simulink model "Pump_system_008"  (R2020a)
settings: Solver=VariableStepAuto  StartTime=0.0  StopTime=1000  MaxStep=0.5  RelTol=1e-3  AbsTol=1e-4
libraries: subsea_lib x65, nesl_utility x44
(part 1 of 2)
settings Model: PauseTimes=645  EnablePacing=on  Creator=piosi  LastModifiedBy=piosi
settings SolverCC: AutoScaleAbsTol=off  MaxOrder=2  MaxConsecutiveZCs=10  MaxConsecutiveMinStep=2  ZeroCrossControl=EnableAll  ZeroCrossAlgorithm=Adaptive
settings DebuggingCC: ReadBeforeWriteMsg=DisableAll  WriteAfterWriteMsg=DisableAll  WriteAfterReadMsg=DisableAll  MultiTaskDSMMsg=none  SymbolicDimsDataTypeCodeGenerationDiagnostic=none
settings ModelReferenceCC: UpdateModelReferenceTargets=IfOutOfDate
settings SFSimCC: SFSimEcho=off  CustomCodeUndefinedFunction=UseInterfaceOnly
settings SimscapeCC: SimscapeLogType=all  SimscapeLogSimulationStatistics=on  SimscapeLogDataHistory=10000

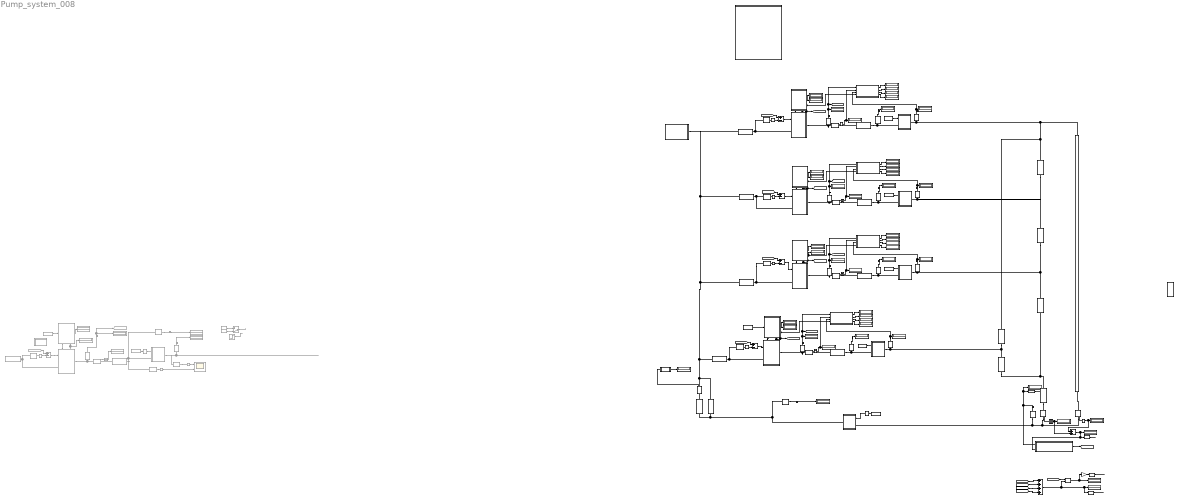
== system Pump_system_008 ==
  note: MANIFOLD
  note: PUMP 801
  note: 1. Find components in the Simscape library .
      | For more information, see Physical Modeling - Blocks .
      | 2. Connect the components to form a physical network.
      | For more information, see Essential Steps for Constructing a Physical Model .
      | 3. Explore simulation results using sscexplore
  note: Simscape Library Resources
  note: PUMP 802
  note: PUMP 803
  note: PUMP 805
  note: PUMP 805
  Add : Sum
  Add1 : Sum  Inputs=++++
  Butterfly valve Z011 : Subsystem
      mask Display: image('D:\CUvalley\Edycja 2\Dane katalogowe\Z-011.png'); % Use "Edit Image" on toolstrip to change.
  Butterfly valve Z1 : Subsystem
      mask Display: image('D:\CUvalley\Edycja 2\Dane katalogowe\Z-011.png'); % Use "Edit Image" on toolstrip to change.
  Butterfly valve Z2 : Subsystem
      mask Display: image('D:\CUvalley\Edycja 2\Dane katalogowe\Z-011.png'); % Use "Edit Image" on toolstrip to change.
  Butterfly valve Z4 : Subsystem
      mask Display: image('D:\CUvalley\Edycja 2\Dane katalogowe\Z-011.png'); % Use "Edit Image" on toolstrip to change.
  Butterfly valve Z5 : Subsystem  Commented=on
      mask Display: image('D:\CUvalley\Edycja 2\Dane katalogowe\Z-011.png'); % Use "Edit Image" on toolstrip to change.
  Constant1 : Constant  Commented=on  Value=0
  Constant2 : Constant  Commented=on
  Display{,1..17,19,21..40,43..51} (48 alike) : Display
      settings: Decimation=2
  Display{52..57} (6 alike) : Display  Commented=on
      settings: Decimation=2
  Divide : Product  Inputs=*/
  From7 : From  Commented=on  GotoTag=p_pump5
  Gain2 : Gain  Gain=100
  Goto10 : Goto  Commented=on  GotoTag=p_pump5
  Hydraulic Pipeline{1,4,10,13} (4 alike) : subsea_lib/Lines/Hydraulic Pipeline  ss_location=true  on_seabed=false  d_in=350 mm  D_out=370 mm  length=10 m  roughness=15e-6 m  Re_lam=2000  Re_turb=4000  wall_type=true  p_init=.101 bar  Young_modulus=5 GPa  time_const=0.01 s  k_sh=1.4
      settings: SourceProductName=Subsea  InternalSimscapePortConfiguration="{\"Bottom\":[],\"Left\":[{\"id\":\"A\",\"label\":\"A\",\"type\":\"subsea.ss_hydraulic\"}],\"Right\":[{\"id\":\"B\",\"label\":\"B\",\"type\":\"subsea.ss_hydraulic\"}],\"Top\":[]}"
  Hydraulic Pipeline{3,5,11,19} (4 alike) : subsea_lib/Lines/Hydraulic Pipeline  ss_location=true  on_seabed=false  d_in=300 mm  D_out=320 mm  length=2 m  roughness=15e-6 m  Re_lam=2000  Re_turb=4000  wall_type=true  p_init=0.1 bar  Young_modulus=195 GPa  time_const=0.01 s  k_sh=1.4
      settings: SourceProductName=Subsea  InternalSimscapePortConfiguration="{\"Bottom\":[],\"Left\":[{\"id\":\"A\",\"label\":\"A\",\"type\":\"subsea.ss_hydraulic\"}],\"Right\":[{\"id\":\"B\",\"label\":\"B\",\"type\":\"subsea.ss_hydraulic\"}],\"Top\":[]}"
  Hydraulic Pipeline12 : subsea_lib/Lines/Hydraulic Pipeline  Commented=on  ss_location=true  on_seabed=false  d_in=350 mm  D_out=370 mm  length=10 m  roughness=15e-6 m  Re_lam=2000  Re_turb=4000  wall_type=true  p_init=.101 bar  Young_modulus=5 GPa  time_const=0.01 s  k_sh=1.4
      settings: SourceProductName=Subsea  InternalSimscapePortConfiguration="{\"Bottom\":[],\"Left\":[{\"id\":\"A\",\"label\":\"A\",\"type\":\"subsea.ss_hydraulic\"}],\"Right\":[{\"id\":\"B\",\"label\":\"B\",\"type\":\"subsea.ss_hydraulic\"}],\"Top\":[]}"
  Hydraulic Pipeline14 : subsea_lib/Lines/Hydraulic Pipeline  ss_location=true  on_seabed=false  d_in=500 mm  D_out=520 mm  length=150 m  roughness=15e-6 m  Re_lam=2000  Re_turb=4000  wall_type=true  p_init=0.1 bar  Young_modulus=6 GPa  time_const=0.01 s  k_sh=1.4
      settings: SourceProductName=Subsea  InternalSimscapePortConfiguration="{\"Bottom\":[],\"Left\":[{\"id\":\"A\",\"label\":\"A\",\"type\":\"subsea.ss_hydraulic\"}],\"Right\":[{\"id\":\"B\",\"label\":\"B\",\"type\":\"subsea.ss_hydraulic\"}],\"Top\":[]}"
  Hydraulic Pipeline15 : subsea_lib/Lines/Hydraulic Pipeline  Commented=on  ss_location=true  on_seabed=false  d_in=300 mm  D_out=320 mm  length=2 m  roughness=15e-6 m  Re_lam=2000  Re_turb=4000  wall_type=true  p_init=0.1 bar  Young_modulus=195 GPa  time_const=0.01 s  k_sh=1.4
      settings: SourceProductName=Subsea  InternalSimscapePortConfiguration="{\"Bottom\":[],\"Left\":[{\"id\":\"A\",\"label\":\"A\",\"type\":\"subsea.ss_hydraulic\"}],\"Right\":[{\"id\":\"B\",\"label\":\"B\",\"type\":\"subsea.ss_hydraulic\"}],\"Top\":[]}"
  Hydraulic Pipeline{6..7,16..17} (4 alike) : subsea_lib/Lines/Hydraulic Pipeline  ss_location=true  on_seabed=false  d_in=500 mm  D_out=520 mm  length=5 m  roughness=15e-6 m  Re_lam=2000  Re_turb=4000  wall_type=true  p_init=0.1 bar  Young_modulus=6 GPa  time_const=0.01 s  k_sh=1.4
      settings: SourceProductName=Subsea  InternalSimscapePortConfiguration="{\"Bottom\":[],\"Left\":[{\"id\":\"A\",\"label\":\"A\",\"type\":\"subsea.ss_hydraulic\"}],\"Right\":[{\"id\":\"B\",\"label\":\"B\",\"type\":\"subsea.ss_hydraulic\"}],\"Top\":[]}"
  Hydraulic Pipeline18 : subsea_lib/Lines/Hydraulic Pipeline  ss_location=true  on_seabed=false  d_in=500 mm  D_out=520 mm  length=20 m  roughness=15e-6 m  Re_lam=2000  Re_turb=4000  wall_type=true  p_init=0.1 bar  Young_modulus=6 GPa  time_const=0.01 s  k_sh=1.4
      settings: SourceProductName=Subsea  InternalSimscapePortConfiguration="{\"Bottom\":[],\"Left\":[{\"id\":\"A\",\"label\":\"A\",\"type\":\"subsea.ss_hydraulic\"}],\"Right\":[{\"id\":\"B\",\"label\":\"B\",\"type\":\"subsea.ss_hydraulic\"}],\"Top\":[]}"
  Hydraulic Pipeline2 : subsea_lib/Lines/Hydraulic Pipeline  ss_location=true  on_seabed=false  d_in=500 mm  D_out=520 mm  length=10 m  roughness=15e-6 m  Re_lam=2000  Re_turb=4000  wall_type=true  p_init=0.1 bar  Young_modulus=6 GPa  time_const=0.01 s  k_sh=1.4
      settings: SourceProductName=Subsea  InternalSimscapePortConfiguration="{\"Bottom\":[],\"Left\":[{\"id\":\"A\",\"label\":\"A\",\"type\":\"subsea.ss_hydraulic\"}],\"Right\":[{\"id\":\"B\",\"label\":\"B\",\"type\":\"subsea.ss_hydraulic\"}],\"Top\":[]}"
  Hydraulic Pipeline20 : subsea_lib/Lines/Hydraulic Pipeline  ss_location=true  on_seabed=false  d_in=500 mm  D_out=520 mm  length=20 m  roughness=15e-6 m  Re_lam=2000  Re_turb=4000  wall_type=true  p_init=0.1 bar  Young_modulus=6 GPa  time_const=0.01 s  k_sh=1.4
      settings: SourceProductName=Subsea  InternalSimscapePortConfiguration="{\"Bottom\":[],\"Left\":[{\"id\":\"A\",\"label\":\"A\",\"type\":\"subsea.ss_hydraulic\"}],\"Right\":[{\"id\":\"B\",\"label\":\"B\",\"type\":\"subsea.ss_hydraulic\"}],\"Top\":[]}"
  Hydraulic Pipeline8 : subsea_lib/Lines/Hydraulic Pipeline  ss_location=true  on_seabed=false  d_in=500 mm  D_out=520 mm  length=30 m  roughness=15e-6 m  Re_lam=2000  Re_turb=4000  wall_type=true  p_init=0.1 bar  Young_modulus=6 GPa  time_const=0.01 s  k_sh=1.4
      settings: SourceProductName=Subsea  InternalSimscapePortConfiguration="{\"Bottom\":[],\"Left\":[{\"id\":\"A\",\"label\":\"A\",\"type\":\"subsea.ss_hydraulic\"}],\"Right\":[{\"id\":\"B\",\"label\":\"B\",\"type\":\"subsea.ss_hydraulic\"}],\"Top\":[]}"
  Hydraulic Pipeline9 : subsea_lib/Lines/Hydraulic Pipeline  ss_location=true  on_seabed=false  d_in=500 mm  D_out=520 mm  length=150 m  roughness=15e-6 m  Re_lam=2000  Re_turb=4000  wall_type=true  p_init=0.1 bar  Young_modulus=6 GPa  time_const=0.01 s  k_sh=1.4
      settings: SourceProductName=Subsea  InternalSimscapePortConfiguration="{\"Bottom\":[],\"Left\":[{\"id\":\"A\",\"label\":\"A\",\"type\":\"subsea.ss_hydraulic\"}],\"Right\":[{\"id\":\"B\",\"label\":\"B\",\"type\":\"subsea.ss_hydraulic\"}],\"Top\":[]}"
  Manual Switch1 : ManualSwitch  Commented=on  CurrentSetting=0
  Opening angle : Constant  Value=86.5
  Opening angle1 : Constant  Value=31
  Opening angle2 : Constant  Value=31.5
  Opening angle3 : Constant  Value=35
  Opening angle5 : Constant  Value=90
  Opening angle6 : Constant  Commented=on  Value=90
  PS-Simulink Converter{1..15,22,25..26} (18 alike) : nesl_utility/PS-Simulink Converter  PhysicalDomain=network_engine_domain  SubClassName=ps_output  LeftPortType=input  RightPortType=output  PseudoPeriodic=off  Frequencies=[]  Unit=inherit  AffineConversion=off
      settings: SourceProductBaseCode=MT,SS
  PS-Simulink Converter{16..17,27..30} (6 alike) : nesl_utility/PS-Simulink Converter  Commented=on  PhysicalDomain=network_engine_domain  SubClassName=ps_output  LeftPortType=input  RightPortType=output  PseudoPeriodic=off  Frequencies=[]  Unit=inherit  AffineConversion=off
      settings: SourceProductBaseCode=MT,SS
  RPM : Constant  Value=1420
  RPM2 : Constant  Commented=on  Value=1060
  Rate Transition{1..2,4..5} (4 alike) : RateTransition  OutPortSampleTime=1
  Return press1 : Scope  Commented=on  NumInputPorts=2
  Step1 : Step  Commented=on  Time=75  SampleTime=0
  Subsea Hydraulic Flow Rate Sensor{1..4,6..8} (7 alike) : subsea_lib/Sensors/Subsea Hydraulic Flow Rate Sensor
      settings: SourceProductName=Subsea  InternalSimscapePortConfiguration="{\"Bottom\":[],\"Left\":[{\"id\":\"A\",\"label\":\"A\",\"type\":\"subsea.ss_hydraulic\"}],\"Right\":[{\"id\":\"Q\",\"label\":\"Q\",\"type\":\"output\"},{\"id\":\"B\",\"label\":\"B\",\"type\":\"subsea.ss_hydraulic\"},{\"id\":\"M\",\"label\":\"M\",\"type\":\"output\"}],\"Top\":[]}"
  Subsea Hydraulic Flow Rate Sensor9 : subsea_lib/Sensors/Subsea Hydraulic Flow Rate Sensor  Commented=on
      settings: SourceProductName=Subsea  InternalSimscapePortConfiguration="{\"Bottom\":[],\"Left\":[{\"id\":\"A\",\"label\":\"A\",\"type\":\"subsea.ss_hydraulic\"}],\"Right\":[{\"id\":\"Q\",\"label\":\"Q\",\"type\":\"output\"},{\"id\":\"B\",\"label\":\"B\",\"type\":\"subsea.ss_hydraulic\"},{\"id\":\"M\",\"label\":\"M\",\"type\":\"output\"}],\"Top\":[]}"
  Subsea Hydraulic Pressure Gauge{1..15,22,25..26} (18 alike) : subsea_lib/Sensors/Subsea Hydraulic Pressure Gauge
      settings: SourceProductName=Subsea  InternalSimscapePortConfiguration="{\"Bottom\":[],\"Left\":[{\"id\":\"A\",\"label\":\"A\",\"type\":\"subsea.ss_hydraulic\"}],\"Right\":[{\"id\":\"P\",\"label\":\"P\",\"type\":\"output\"}],\"Top\":[]}"
  Subsea Hydraulic Pressure Gauge{16..17,27..30} (6 alike) : subsea_lib/Sensors/Subsea Hydraulic Pressure Gauge  Commented=on
      settings: SourceProductName=Subsea  InternalSimscapePortConfiguration="{\"Bottom\":[],\"Left\":[{\"id\":\"A\",\"label\":\"A\",\"type\":\"subsea.ss_hydraulic\"}],\"Right\":[{\"id\":\"P\",\"label\":\"P\",\"type\":\"output\"}],\"Top\":[]}"
  Subsystem : Subsystem
      mask Help: web(htmlFile)
  Subsystem1 : Subsystem
      mask Help: web(htmlFile)
  Subsystem10 : Subsystem
  Subsystem11 : Subsystem
  Subsystem12 : Subsystem
      settings: PortSchema="{\"entries\":[{\"content\":{\"sides\":[{\"content\":{\"connectorIds\":[\"In1\",\"LConn1\"]},\"type\":\"ConnectorPlacement.EquallySpacedRectSide\",\"uuid\":\"b08fe6bd-5385-402a-970e-44a5082313f0\"},{\"content\":{\"connectorIds\":[\"RConn1\"],\"side\":\"RIGHT\"},\"type\":\"ConnectorPlacement.EquallySpacedRectSide\",\"uuid\":\"0f55c765-16c9-4350-ba94-56cdb1c15382\"},{\"content\":{\"connectorIds\":[\"In2\",\"Out1\"],\"side\":\"TOP\"},\"type\":\"ConnectorPlacement.EquallySpacedRectSide\",\"uuid\":\"97e0110d-4c8c-4a3d-88de-aced2dd12bff\"}]},\"type\":\"ConnectorPlacement.EquallySpacedConnector\",\"uuid\":\"8cd8dc67-fa80-4707-b9c2-3021d4be2722\"}],\"packageUris\":[\"http://schema.mathworks.com/mf0/Connector/19700101\"],\"version\":\"1.0\"}"
      mask Display: image('D:\CUvalley\Edycja 2\Dane katalogowe\pump.png'); % Use "Edit Image" on toolstrip to change.
  Subsystem15 : Subsystem
      mask Help: web(htmlFile)
  Subsystem16 : Subsystem
  Subsystem17 : Subsystem
      settings: PortSchema="{\"entries\":[{\"content\":{\"sides\":[{\"content\":{\"connectorIds\":[]},\"type\":\"ConnectorPlacement.EquallySpacedRectSide\",\"uuid\":\"50845c6e-5ce5-420a-b8f7-3857dcaa504f\"},{\"content\":{\"connectorIds\":[\"Out1\"],\"side\":\"RIGHT\"},\"type\":\"ConnectorPlacement.EquallySpacedRectSide\",\"uuid\":\"cc8e2bf6-8706-4441-b0e4-e4ffa0c8e657\"},{\"content\":{\"connectorIds\":[],\"side\":\"TOP\"},\"type\":\"ConnectorPlacement.EquallySpacedRectSide\",\"uuid\":\"432846fe-ee00-4555-9242-668b3d13e87b\"},{\"content\":{\"connectorIds\":[\"Out2\",\"In1\"],\"side\":\"BOTTOM\"},\"type\":\"ConnectorPlacement.EquallySpacedRectSide\",\"uuid\":\"d8599d27-832c-4fe7-937c-70c6baa9b63a\"}]},\"type\":\"ConnectorPlacement.EquallySpacedConnector\",\"uuid\":\"f9d9813c-d2f5-4a73-8d0c-3cbf729a4c7d\"}],\"packageUris\":[\"http://schema.mathworks.com/mf0/Connector/19700101\"],\"version\":\"1.0\"}"
      mask Display: image('D:\CUvalley\Edycja 2\Dane katalogowe\motor.png'); % Use "Edit Image" on toolstrip to change.
  Subsystem18 : Subsystem
  Subsystem2 : Subsystem
      settings: PortSchema="{\"entries\":[{\"content\":{\"sides\":[{\"content\":{\"connectorIds\":[]},\"type\":\"ConnectorPlacement.EquallySpacedRectSide\",\"uuid\":\"50845c6e-5ce5-420a-b8f7-3857dcaa504f\"},{\"content\":{\"connectorIds\":[\"Out1\"],\"side\":\"RIGHT\"},\"type\":\"ConnectorPlacement.EquallySpacedRectSide\",\"uuid\":\"cc8e2bf6-8706-4441-b0e4-e4ffa0c8e657\"},{\"content\":{\"connectorIds\":[],\"side\":\"TOP\"},\"type\":\"ConnectorPlacement.EquallySpacedRectSide\",\"uuid\":\"432846fe-ee00-4555-9242-668b3d13e87b\"},{\"content\":{\"connectorIds\":[\"Out2\",\"In1\"],\"side\":\"BOTTOM\"},\"type\":\"ConnectorPlacement.EquallySpacedRectSide\",\"uuid\":\"d8599d27-832c-4fe7-937c-70c6baa9b63a\"}]},\"type\":\"ConnectorPlacement.EquallySpacedConnector\",\"uuid\":\"f9d9813c-d2f5-4a73-8d0c-3cbf729a4c7d\"}],\"packageUris\":[\"http://schema.mathworks.com/mf0/Connector/19700101\"],\"version\":\"1.0\"}"
      mask Display: image('D:\CUvalley\Edycja 2\Dane katalogowe\motor.png'); % Use "Edit Image" on toolstrip to change.
  Subsystem20 : Subsystem
      settings: PortSchema="{\"entries\":[{\"content\":{\"sides\":[{\"content\":{\"connectorIds\":[\"In1\"]},\"type\":\"ConnectorPlacement.EquallySpacedRectSide\",\"uuid\":\"50845c6e-5ce5-420a-b8f7-3857dcaa504f\"},{\"content\":{\"connectorIds\":[\"Out1\"],\"side\":\"RIGHT\"},\"type\":\"ConnectorPlacement.EquallySpacedRectSide\",\"uuid\":\"cc8e2bf6-8706-4441-b0e4-e4ffa0c8e657\"},{\"content\":{\"connectorIds\":[],\"side\":\"TOP\"},\"type\":\"ConnectorPlacement.EquallySpacedRectSide\",\"uuid\":\"432846fe-ee00-4555-9242-668b3d13e87b\"},{\"content\":{\"connectorIds\":[\"Out2\",\"In2\"],\"side\":\"BOTTOM\"},\"type\":\"ConnectorPlacement.EquallySpacedRectSide\",\"uuid\":\"d8599d27-832c-4fe7-937c-70c6baa9b63a\"}]},\"type\":\"ConnectorPlacement.EquallySpacedConnector\",\"uuid\":\"f9d9813c-d2f5-4a73-8d0c-3cbf729a4c7d\"}],\"packageUris\":[\"http://schema.mathworks.com/mf0/Connector/19700101\"],\"version\":\"1.0\"}"
      mask Display: image('D:\CUvalley\Edycja 2\Dane katalogowe\motor.png'); % Use "Edit Image" on toolstrip to change.
  Subsystem21 : Subsystem
      settings: PortSchema="{\"entries\":[{\"content\":{\"sides\":[{\"content\":{\"connectorIds\":[\"In1\",\"LConn1\"]},\"type\":\"ConnectorPlacement.EquallySpacedRectSide\",\"uuid\":\"00f4933c-19dc-4ef0-b562-805df71cc93e\"},{\"content\":{\"connectorIds\":[\"RConn1\"],\"side\":\"RIGHT\"},\"type\":\"ConnectorPlacement.EquallySpacedRectSide\",\"uuid\":\"f2b6827a-b045-4dc6-90cf-bf3b3d1f0ae2\"},{\"content\":{\"connectorIds\":[\"In2\",\"Out1\"],\"side\":\"TOP\"},\"type\":\"ConnectorPlacement.EquallySpacedRectSide\",\"uuid\":\"f6d9d097-f0fb-4eaa-90ee-cdbf5da64074\"}]},\"type\":\"ConnectorPlacement.EquallySpacedConnector\",\"uuid\":\"0ce8892d-dfe0-43a9-b340-454127903a9f\"}],\"packageUris\":[\"http://schema.mathworks.com/mf0/Connector/19700101\"],\"version\":\"1.0\"}"
      mask Display: image('D:\CUvalley\Edycja 2\Dane katalogowe\pump.png'); % Use "Edit Image" on toolstrip to change.
  Subsystem22 : Subsystem
  Subsystem23 : Subsystem  Commented=on
      mask Help: web(htmlFile)
  Subsystem24 : Subsystem
      mask Help: web(htmlFile)
  Subsystem25 : Subsystem  Commented=on
      settings: PortSchema="{\"entries\":[{\"content\":{\"sides\":[{\"content\":{\"connectorIds\":[\"In1\",\"LConn1\"]},\"type\":\"ConnectorPlacement.EquallySpacedRectSide\",\"uuid\":\"00f4933c-19dc-4ef0-b562-805df71cc93e\"},{\"content\":{\"connectorIds\":[\"RConn1\"],\"side\":\"RIGHT\"},\"type\":\"ConnectorPlacement.EquallySpacedRectSide\",\"uuid\":\"f2b6827a-b045-4dc6-90cf-bf3b3d1f0ae2\"},{\"content\":{\"connectorIds\":[\"In2\",\"Out1\"],\"side\":\"TOP\"},\"type\":\"ConnectorPlacement.EquallySpacedRectSide\",\"uuid\":\"f6d9d097-f0fb-4eaa-90ee-cdbf5da64074\"}]},\"type\":\"ConnectorPlacement.EquallySpacedConnector\",\"uuid\":\"0ce8892d-dfe0-43a9-b340-454127903a9f\"}],\"packageUris\":[\"http://schema.mathworks.com/mf0/Connector/19700101\"],\"version\":\"1.0\"}"
      mask Display: image('D:\CUvalley\Edycja 2\Dane katalogowe\pump.png'); % Use "Edit Image" on toolstrip to change.
  Subsystem26 : Subsystem  Commented=on
  Subsystem27 : Subsystem  Commented=on
      settings: PortSchema="{\"entries\":[{\"content\":{\"sides\":[{\"content\":{\"connectorIds\":[\"In1\"]},\"type\":\"ConnectorPlacement.EquallySpacedRectSide\",\"uuid\":\"50845c6e-5ce5-420a-b8f7-3857dcaa504f\"},{\"content\":{\"connectorIds\":[\"Out1\"],\"side\":\"RIGHT\"},\"type\":\"ConnectorPlacement.EquallySpacedRectSide\",\"uuid\":\"cc8e2bf6-8706-4441-b0e4-e4ffa0c8e657\"},{\"content\":{\"connectorIds\":[],\"side\":\"TOP\"},\"type\":\"ConnectorPlacement.EquallySpacedRectSide\",\"uuid\":\"432846fe-ee00-4555-9242-668b3d13e87b\"},{\"content\":{\"connectorIds\":[\"Out2\",\"In2\"],\"side\":\"BOTTOM\"},\"type\":\"ConnectorPlacement.EquallySpacedRectSide\",\"uuid\":\"d8599d27-832c-4fe7-937c-70c6baa9b63a\"}]},\"type\":\"ConnectorPlacement.EquallySpacedConnector\",\"uuid\":\"f9d9813c-d2f5-4a73-8d0c-3cbf729a4c7d\"}],\"packageUris\":[\"http://schema.mathworks.com/mf0/Connector/19700101\"],\"version\":\"1.0\"}"
      mask Display: image('D:\CUvalley\Edycja 2\Dane katalogowe\motor.png'); % Use "Edit Image" on toolstrip to change.
  Subsystem3 : Subsystem
      mask Help: web(htmlFile)
  Subsystem4 : Subsystem
      mask Help: web(htmlFile)
  Subsystem5 : Subsystem
      settings: PortSchema="{\"entries\":[{\"content\":{\"sides\":[{\"content\":{\"connectorIds\":[\"In1\",\"LConn1\"]},\"type\":\"ConnectorPlacement.EquallySpacedRectSide\",\"uuid\":\"b08fe6bd-5385-402a-970e-44a5082313f0\"},{\"content\":{\"connectorIds\":[\"RConn1\"],\"side\":\"RIGHT\"},\"type\":\"ConnectorPlacement.EquallySpacedRectSide\",\"uuid\":\"0f55c765-16c9-4350-ba94-56cdb1c15382\"},{\"content\":{\"connectorIds\":[\"In2\",\"Out1\"],\"side\":\"TOP\"},\"type\":\"ConnectorPlacement.EquallySpacedRectSide\",\"uuid\":\"97e0110d-4c8c-4a3d-88de-aced2dd12bff\"}]},\"type\":\"ConnectorPlacement.EquallySpacedConnector\",\"uuid\":\"8cd8dc67-fa80-4707-b9c2-3021d4be2722\"}],\"packageUris\":[\"http://schema.mathworks.com/mf0/Connector/19700101\"],\"version\":\"1.0\"}"
      mask Display: image('D:\CUvalley\Edycja 2\Dane katalogowe\pump.png'); % Use "Edit Image" on toolstrip to change.
  Subsystem6 : Subsystem
  Subsystem7 : Subsystem
      settings: PortSchema="{\"entries\":[{\"content\":{\"sides\":[{\"content\":{\"connectorIds\":[]},\"type\":\"ConnectorPlacement.EquallySpacedRectSide\",\"uuid\":\"50845c6e-5ce5-420a-b8f7-3857dcaa504f\"},{\"content\":{\"connectorIds\":[\"Out1\"],\"side\":\"RIGHT\"},\"type\":\"ConnectorPlacement.EquallySpacedRectSide\",\"uuid\":\"cc8e2bf6-8706-4441-b0e4-e4ffa0c8e657\"},{\"content\":{\"connectorIds\":[],\"side\":\"TOP\"},\"type\":\"ConnectorPlacement.EquallySpacedRectSide\",\"uuid\":\"432846fe-ee00-4555-9242-668b3d13e87b\"},{\"content\":{\"connectorIds\":[\"Out2\",\"In1\"],\"side\":\"BOTTOM\"},\"type\":\"ConnectorPlacement.EquallySpacedRectSide\",\"uuid\":\"d8599d27-832c-4fe7-937c-70c6baa9b63a\"}]},\"type\":\"ConnectorPlacement.EquallySpacedConnector\",\"uuid\":\"f9d9813c-d2f5-4a73-8d0c-3cbf729a4c7d\"}],\"packageUris\":[\"http://schema.mathworks.com/mf0/Connector/19700101\"],\"version\":\"1.0\"}"
      mask Display: image('D:\CUvalley\Edycja 2\Dane katalogowe\motor.png'); % Use "Edit Image" on toolstrip to change.
  Subsystem8 : Subsystem
      mask Help: web(htmlFile)
  Subsystem9 : Subsystem
      settings: PortSchema="{\"entries\":[{\"content\":{\"sides\":[{\"content\":{\"connectorIds\":[\"In1\",\"LConn1\"]},\"type\":\"ConnectorPlacement.EquallySpacedRectSide\",\"uuid\":\"b08fe6bd-5385-402a-970e-44a5082313f0\"},{\"content\":{\"connectorIds\":[\"RConn1\"],\"side\":\"RIGHT\"},\"type\":\"ConnectorPlacement.EquallySpacedRectSide\",\"uuid\":\"0f55c765-16c9-4350-ba94-56cdb1c15382\"},{\"content\":{\"connectorIds\":[\"In2\",\"Out1\"],\"side\":\"TOP\"},\"type\":\"ConnectorPlacement.EquallySpacedRectSide\",\"uuid\":\"97e0110d-4c8c-4a3d-88de-aced2dd12bff\"}]},\"type\":\"ConnectorPlacement.EquallySpacedConnector\",\"uuid\":\"8cd8dc67-fa80-4707-b9c2-3021d4be2722\"}],\"packageUris\":[\"http://schema.mathworks.com/mf0/Connector/19700101\"],\"version\":\"1.0\"}"
      mask Display: image('D:\CUvalley\Edycja 2\Dane katalogowe\pump.png'); % Use "Edit Image" on toolstrip to change.
  Subtract{1..3,5} (4 alike) : Sum  Inputs=+-
  Subtract6 : Sum  Commented=on  Inputs=+-
  Tank : Subsystem  AncestorBlock=comp_library/Tank
      mask Display: image('reservoir.bmp'); % Use "Edit Image" on toolstrip to change.
  Transfer Fcn1 : TransferFcn  Commented=on  Denominator=[0.5/5 1]
  Transfer Fcn4 : TransferFcn  Denominator=[0.5/5 1]
  restriction : Subsystem
      mask Display: image('D:\CUvalley\Edycja 2\Dane katalogowe\Z-011.png'); % Use "Edit Image" on toolstrip to change.
  wires:
  Subsystem/1(Q m3/h) -> Add/2, Display/1
  [p_pump1] -> Subtract2/1
  PS-Simulink Converter22/1 -> Subtract2/2
  Subtract2/1 -> Subsystem12/1(Pump p)
  Subsystem1/1(Q m3/h) -> Subsystem16/2(In4), Display1/1  "flow_pump1"
  PS-Simulink Converter1/1 -> Subsystem16/1(Pump pressure), [p_pump1], Display2/1  "p_pump1"
  Opening angle1/1 -> Butterfly valve Z011/1(In1)
  Subsystem12/1(Power) -> Subsystem2/1(Power), [power_motor1], Display3/1, Subsystem16/4(In3)  "power_motor1"
  Subsystem2/2(Out1) -> Subsystem12/2(RPM)
  PS-Simulink Converter2/1 -> Display5/1
  Subsystem3/1(Q m3/h) -> Display4/1
  Transfer Fcn4/1 -> restriction/1(In1)
  Opening angle/1 -> Transfer Fcn4/1
  PS-Simulink Converter26/1 -> Display23/1
  Subsystem15/1(Q m3/h) -> Add/1, Display24/1
  Subsystem2/1(current) -> Display26/1  "Current_motor1"
  PS-Simulink Converter3/1 -> Subsystem16/3(In2), Display6/1
  Subsystem16/1(Hyd Power pump) -> Display27/1
  Subsystem16/2(Hyd Power pipeline) -> Display28/1
  Subsystem16/3(Hyd Eff pump) -> Display29/1
  Subsystem16/4(Hyd Eff pipeline) -> Display30/1  "hyd_eff_pipe1"
  Subsystem6/4(Hyd Eff pipeline) -> Display33/1  "hyd_eff_pipe2"
  Subsystem6/3(Hyd Eff pump) -> Display31/1
  Subsystem6/2(Hyd Power pipeline) -> Display11/1
  Subsystem6/1(Hyd Power pump) -> Display10/1
  PS-Simulink Converter7/1 -> Display35/1, Subsystem6/3(In2)
  Subsystem17/1(current) -> Display9/1  "Current_motor1"
  PS-Simulink Converter5/1 -> Display34/1
  Subsystem17/2(Out1) -> Subsystem5/2(RPM)
  Subsystem5/1(Power) -> Subsystem6/4(In3), Display32/1, [power_motor2], Subsystem17/1(Power)  "power_motor2"
  Opening angle2/1 -> Butterfly valve Z1/1(In1)
  PS-Simulink Converter4/1 -> Display8/1, [p_pump2], Subsystem6/1(Pump pressure)  "p_pump2"
  Subsystem4/1(Q m3/h) -> Display7/1, Subsystem6/2(In4)  "flow_pump2"
  Subtract1/1 -> Subsystem5/1(Pump p)
  PS-Simulink Converter6/1 -> Subtract1/2
  [p_pump2] -> Subtract1/1
  Subsystem18/2(Hyd Power pipeline) -> Display13/1
  Subsystem18/3(Hyd Eff pump) -> Display14/1
  Subsystem18/4(Hyd Eff pipeline) -> Display16/1  "hyd_eff_pipe3"
  PS-Simulink Converter9/1 -> Display36/1
  Subsystem7/1(current) -> Display40/1  "Current_motor1"
  PS-Simulink Converter11/1 -> Display37/1, Subsystem18/3(In2)
  Subsystem18/1(Hyd Power pump) -> Display12/1
  PS-Simulink Converter10/1 -> Subtract3/2
  [p_pump3] -> Subtract3/1
  Subtract3/1 -> Subsystem9/1(Pump p)
  Subsystem8/1(Q m3/h) -> Display38/1, Subsystem18/2(In4)  "flow_pump3"
  Subsystem9/1(Power) -> Subsystem18/4(In3), Display15/1, [power_motor3], Subsystem7/1(Power)  "power_motor3"
  Opening angle3/1 -> Butterfly valve Z2/1(In1)
  PS-Simulink Converter8/1 -> Display39/1, [p_pump3], Subsystem18/1(Pump pressure)  "p_pump3"
  Subsystem7/2(Out1) -> Subsystem9/2(RPM)
  RPM/1 -> Subsystem20/1(In1)
  PS-Simulink Converter14/1 -> Display50/1, [p_pump5], Subsystem22/1(Pump pressure)  "p_pump5"
  Subsystem21/1(Power) -> Subsystem22/4(In3), Display45/1, [power_motor5], Subsystem20/2(Power)  "power_motor5"
  Subsystem24/1(Q m3/h) -> Display49/1, Subsystem22/2(In4)  "flow_pump5"
  [p_pump5] -> Subtract5/1
  Subsystem22/1(Hyd Power pump) -> Display21/1
  PS-Simulink Converter13/1 -> Display48/1, Subsystem22/3(In2)
  Subsystem20/1(current) -> Display51/1  "Current_motor5"
  PS-Simulink Converter15/1 -> Display47/1
  Subsystem22/4(Hyd Eff pipeline) -> Display46/1  "hyd_eff_pipe5"
  Opening angle5/1 -> Butterfly valve Z4/1(In1)
  Subsystem20/2(Out1) -> Subsystem21/2(RPM)
  Subtract5/1 -> Subsystem21/1(Pump p)
  Subsystem22/3(Hyd Eff pump) -> Display44/1
  PS-Simulink Converter12/1 -> Subtract5/2
  Subsystem22/2(Hyd Power pipeline) -> Display43/1
  Subsystem27/2(Out1) -> Subsystem25/2(RPM)
  Manual Switch1/1 -> ?
  Step1/1 -> ?
  Constant2/1 -> Manual Switch1/1
  Constant1/1 -> Manual Switch1/2
  From7/1 -> Subtract6/1
  Opening angle6/1 -> Transfer Fcn1/1
  PS-Simulink Converter29/1 -> Subtract6/2
  RPM2/1 -> Subsystem27/1(In1)
  PS-Simulink Converter16/1 -> Return press1/1
  PS-Simulink Converter27/1 -> Return press1/2
  Subtract6/1 -> Subsystem25/1(Pump p)
  PS-Simulink Converter28/1 -> Display52/1
  Transfer Fcn1/1 -> Butterfly valve Z5/1(In1)
  Subsystem23/1(Q m3/h) -> Display54/1  "flow_pump5"
  PS-Simulink Converter30/1 -> Display53/1
  Subsystem27/1(current) -> Display57/1  "Current_motor5"
  Subsystem25/1(Power) -> Display56/1, Subsystem27/2(Power)  "power_motor5"
  PS-Simulink Converter17/1 -> Display55/1, Goto10/1  "Pump pressure"
  [power_motor3] -> Add1/3
  [power_motor2] -> Add1/2
  [power_motor5] -> Add1/4
  [power_motor1] -> Add1/1
  Add1/1 -> Display17/1, Rate Transition2/1, Divide/2  "power_motor_total"
  PS-Simulink Converter25/1 -> Subsystem10/1(In1), Display22/1, Rate Transition4/1
  [power_pipeline] -> Divide/1
  Divide/1 -> Gain2/1, Display19/1  "eff_total"
  Rate Transition1/1 -> ?  "Efficiency total"
  Rate Transition2/1 -> ?  "Motor power total"
  Rate Transition4/1 -> ?  "Manifold pressure"
  Rate Transition5/1 -> ?  "Manifold flow"
  Add/1 -> Display25/1, Subsystem10/2(power_pipeline), Rate Transition5/1  "power_pipeline"
  Gain2/1 -> Rate Transition1/1
  Subsystem10/1(power_pipeline1) -> [power_pipeline]
  connections:
  Hydraulic Pipeline13/RConn1 -- Butterfly valve Z011/LConn1 -- Subsea Hydraulic Pressure Gauge2/LConn1
  Subsystem/LConn1 -- Subsea Hydraulic Flow Rate Sensor1/RConn1
  Subsea Hydraulic Flow Rate Sensor4/RConn1 -- Subsystem3/LConn1
  Subsea Hydraulic Flow Rate Sensor6/RConn1 -- Subsystem1/LConn1
  Hydraulic Pipeline13/LConn1 -- Subsea Hydraulic Flow Rate Sensor6/RConn2
  Hydraulic Pipeline19/LConn1 -- Hydraulic Pipeline11/LConn1 -- Hydraulic Pipeline9/LConn1 -- Subsea Hydraulic Flow Rate Sensor4/RConn2 -- Hydraulic Pipeline5/LConn1 -- Tank/LConn1 -- Hydraulic Pipeline3/LConn1
  Subsystem12/RConn1 -- Subsea Hydraulic Pressure Gauge1/LConn1 -- Subsea Hydraulic Flow Rate Sensor6/LConn1
  Subsystem12/LConn1 -- Subsea Hydraulic Pressure Gauge22/LConn1 -- Hydraulic Pipeline19/RConn1
  Hydraulic Pipeline14/LConn1 -- Subsea Hydraulic Flow Rate Sensor4/LConn1
  Subsea Hydraulic Pressure Gauge22/RConn1 -- PS-Simulink Converter22/LConn1
  Subsea Hydraulic Flow Rate Sensor1/RConn2 -- Subsea Hydraulic Flow Rate Sensor7/RConn2 -- Subsea Hydraulic Pressure Gauge25/LConn1 -- restriction/LConn1
  Butterfly valve Z4/RConn1 -- Hydraulic Pipeline20/LConn1 -- Hydraulic Pipeline18/LConn1 -- Subsea Hydraulic Pressure Gauge13/LConn1
  Subsea Hydraulic Pressure Gauge1/RConn1 -- PS-Simulink Converter1/LConn1
  Subsea Hydraulic Pressure Gauge2/RConn1 -- PS-Simulink Converter2/LConn1
  Subsea Hydraulic Pressure Gauge3/RConn1 -- PS-Simulink Converter3/LConn1
  Hydraulic Pipeline2/RConn1 -- Subsea Hydraulic Flow Rate Sensor1/LConn1
  restriction/RConn1 -- Subsea Hydraulic Pressure Gauge26/LConn1 -- Hydraulic Pipeline9/RConn1 -- Hydraulic Pipeline14/RConn1
  Subsea Hydraulic Pressure Gauge25/RConn1 -- PS-Simulink Converter25/LConn1
  Subsea Hydraulic Pressure Gauge26/RConn1 -- PS-Simulink Converter26/LConn1
  Subsystem15/LConn1 -- Subsea Hydraulic Flow Rate Sensor7/RConn1
  Subsea Hydraulic Flow Rate Sensor7/LConn1 -- Hydraulic Pipeline8/RConn1
  Butterfly valve Z1/LConn1 -- Subsea Hydraulic Pressure Gauge5/LConn1 -- Hydraulic Pipeline1/RConn1
  Subsystem5/RConn1 -- Subsea Hydraulic Flow Rate Sensor2/LConn1 -- Subsea Hydraulic Pressure Gauge4/LConn1
  Subsea Hydraulic Pressure Gauge6/LConn1 -- Subsystem5/LConn1 -- Hydraulic Pipeline3/RConn1
  Subsea Hydraulic Pressure Gauge5/RConn1 -- PS-Simulink Converter5/LConn1
  Subsea Hydraulic Pressure Gauge4/RConn1 -- PS-Simulink Converter4/LConn1
  Subsea Hydraulic Pressure Gauge7/RConn1 -- PS-Simulink Converter7/LConn1
  Hydraulic Pipeline1/LConn1 -- Subsea Hydraulic Flow Rate Sensor2/RConn2
  Subsea Hydraulic Pressure Gauge6/RConn1 -- PS-Simulink Converter6/LConn1
  Subsea Hydraulic Flow Rate Sensor2/RConn1 -- Subsystem4/LConn1
  Butterfly valve Z2/LConn1 -- Subsea Hydraulic Pressure Gauge9/LConn1 -- Hydraulic Pipeline4/RConn1
  Subsea Hydraulic Pressure Gauge10/LConn1 -- Hydraulic Pipeline5/RConn1 -- Subsystem9/LConn1
  Subsystem9/RConn1 -- Subsea Hydraulic Flow Rate Sensor3/LConn1 -- Subsea Hydraulic Pressure Gauge8/LConn1
  Subsea Hydraulic Pressure Gauge10/RConn1 -- PS-Simulink Converter10/LConn1
  Subsea Hydraulic Pressure Gauge9/RConn1 -- PS-Simulink Converter9/LConn1
  Subsea Hydraulic Flow Rate Sensor3/RConn1 -- Subsystem8/LConn1
  Subsea Hydraulic Pressure Gauge11/RConn1 -- PS-Simulink Converter11/LConn1
  Subsea Hydraulic Pressure Gauge8/RConn1 -- PS-Simulink Converter8/LConn1
  Hydraulic Pipeline4/LConn1 -- Subsea Hydraulic Flow Rate Sensor3/RConn2
  Butterfly valve Z4/LConn1 -- Subsea Hydraulic Pressure Gauge15/LConn1 -- Hydraulic Pipeline10/RConn1
  Subsea Hydraulic Pressure Gauge14/LConn1 -- Subsystem21/RConn1 -- Subsea Hydraulic Flow Rate Sensor8/LConn1
  Subsea Hydraulic Pressure Gauge12/LConn1 -- Subsystem21/LConn1 -- Hydraulic Pipeline11/RConn1
  Subsea Hydraulic Pressure Gauge12/RConn1 -- PS-Simulink Converter12/LConn1
  Subsea Hydraulic Pressure Gauge14/RConn1 -- PS-Simulink Converter14/LConn1
  Subsea Hydraulic Pressure Gauge15/RConn1 -- PS-Simulink Converter15/LConn1
  Hydraulic Pipeline10/LConn1 -- Subsea Hydraulic Flow Rate Sensor8/RConn2
  Subsea Hydraulic Flow Rate Sensor8/RConn1 -- Subsystem24/LConn1
  Subsea Hydraulic Pressure Gauge13/RConn1 -- PS-Simulink Converter13/LConn1
  Subsystem25/LConn1 -- Hydraulic Pipeline15/RConn1 -- Subsea Hydraulic Pressure Gauge29/LConn1
  Subsea Hydraulic Pressure Gauge28/LConn1 -- Hydraulic Pipeline12/RConn1 -- Subsea Hydraulic Pressure Gauge27/LConn1 -- Butterfly valve Z5/LConn1
  Subsea Hydraulic Pressure Gauge30/LConn1 -- Subsea Hydraulic Pressure Gauge16/LConn1 -- Butterfly valve Z5/RConn1
  Subsystem25/RConn1 -- Subsea Hydraulic Flow Rate Sensor9/LConn1 -- Subsea Hydraulic Pressure Gauge17/LConn1
  Subsea Hydraulic Pressure Gauge30/RConn1 -- PS-Simulink Converter30/LConn1
  Subsea Hydraulic Pressure Gauge27/RConn1 -- PS-Simulink Converter27/LConn1
  Subsea Hydraulic Pressure Gauge16/RConn1 -- PS-Simulink Converter16/LConn1
  Subsea Hydraulic Pressure Gauge28/RConn1 -- PS-Simulink Converter28/LConn1
  Subsea Hydraulic Flow Rate Sensor9/RConn1 -- Subsystem23/LConn1
  Hydraulic Pipeline12/LConn1 -- Subsea Hydraulic Flow Rate Sensor9/RConn2
  Subsea Hydraulic Pressure Gauge17/RConn1 -- PS-Simulink Converter17/LConn1
  Subsea Hydraulic Pressure Gauge29/RConn1 -- PS-Simulink Converter29/LConn1
  Subsea Hydraulic Pressure Gauge7/LConn1 -- Butterfly valve Z1/RConn1 -- Hydraulic Pipeline17/RConn1 -- Hydraulic Pipeline16/LConn1
  Hydraulic Pipeline16/RConn1 -- Hydraulic Pipeline6/LConn1 -- Subsea Hydraulic Pressure Gauge3/LConn1 -- Butterfly valve Z011/RConn1
  Subsea Hydraulic Pressure Gauge11/LConn1 -- Hydraulic Pipeline20/RConn1 -- Hydraulic Pipeline17/LConn1 -- Hydraulic Pipeline8/LConn1 -- Butterfly valve Z2/RConn1
  Hydraulic Pipeline18/RConn1 -- Hydraulic Pipeline2/LConn1 -- Hydraulic Pipeline6/RConn1

== system Pump_system_008/Butterfly valve Z011 ==
  In1 : Inport
  Rate Transition1 : RateTransition  OutPortSampleTime=1
  Simulink-PS Converter4 : nesl_utility/Simulink-PS Converter  PhysicalDomain=network_engine_domain  SubClassName=ps_input  LeftPortType=input  RightPortType=output  PseudoPeriodic=off  Frequencies=[]  NoiseDistribution=none  NoiseParameters=[]  Unit=m^3/s  AffineConversion=off  FilteringAndDerivatives=provide  SimscapeFilterOrder=1  InputFilterTimeConstant=0.001  UdotUserProvided=0
      settings: SourceProductBaseCode=MT,SS
  Transfer Fcn2 : TransferFcn  Denominator=[0.5/5 1]
  Variable kv Hydraulic Flow Element : subsea_lib/Valves/Variable kv Hydraulic Flow Element  ss_location=true  kv=1/3600 m^3/s  kv_min=1.3e-6 m^3/s  q_specify=off  q_priority=None  q=0 m^3/s  q_nominal_specify=off  q_nominal_unit=m^3/s  q_nominal_value=1  p_specify=off  p_priority=None  p=0 Pa  p_nominal_specify=off  p_nominal_unit=Pa  p_nominal_value=1
      settings: SourceProductName=Subsea  InternalSimscapePortConfiguration="{\"Bottom\":[],\"Left\":[{\"id\":\"CS\",\"label\":\"CS\",\"type\":\"input\"},{\"id\":\"A\",\"label\":\"A\",\"type\":\"subsea.ss_hydraulic\"}],\"Right\":[{\"id\":\"B\",\"label\":\"B\",\"type\":\"subsea.ss_hydraulic\"}],\"Top\":[]}"
  Z-011A DN 350 : Lookup_n-D  NumberOfTableDimensions=1  BreakpointsForDimension1=[0 20 30 40 50 60 70 80 90]  BreakpointsForDimension2=[1:3]  Table=[0 399 488 1070 2110 3590 5480 7760 10400]  InternalRulePriority=Speed  RndMeth=Simplest  InputSameDT=on
  Variable kv Hydraulic Flow Element1 : PMIOPort  Side=Left
  Variable kv Hydraulic Flow Element2 : PMIOPort  Port=2  Side=Right
  wires:
  Z-011A DN 350/1 -> Simulink-PS Converter4/1
  In1/1 -> Rate Transition1/1, Transfer Fcn2/1
  Transfer Fcn2/1 -> Z-011A DN 350/1
  Rate Transition1/1 -> ?  "Valve1 opening"
  connections:
  Variable kv Hydraulic Flow Element/RConn1 -- Variable kv Hydraulic Flow Element2/RConn1
  Simulink-PS Converter4/RConn1 -- Variable kv Hydraulic Flow Element/LConn1
  Variable kv Hydraulic Flow Element/LConn2 -- Variable kv Hydraulic Flow Element1/RConn1

== system Pump_system_008/Butterfly valve Z1 ==
  In1 : Inport
  Rate Transition1 : RateTransition  OutPortSampleTime=1
  Simulink-PS Converter4 : nesl_utility/Simulink-PS Converter  PhysicalDomain=network_engine_domain  SubClassName=ps_input  LeftPortType=input  RightPortType=output  PseudoPeriodic=off  Frequencies=[]  NoiseDistribution=none  NoiseParameters=[]  Unit=m^3/s  AffineConversion=off  FilteringAndDerivatives=provide  SimscapeFilterOrder=1  InputFilterTimeConstant=0.001  UdotUserProvided=0
      settings: SourceProductBaseCode=MT,SS
  Transfer Fcn2 : TransferFcn  Denominator=[0.5/5 1]
  Variable kv Hydraulic Flow Element : subsea_lib/Valves/Variable kv Hydraulic Flow Element  ss_location=true  kv=1/3600 m^3/s  kv_min=1.3e-6 m^3/s  q_specify=off  q_priority=None  q=0 m^3/s  q_nominal_specify=off  q_nominal_unit=m^3/s  q_nominal_value=1  p_specify=off  p_priority=None  p=0 Pa  p_nominal_specify=off  p_nominal_unit=Pa  p_nominal_value=1
      settings: SourceProductName=Subsea  InternalSimscapePortConfiguration="{\"Bottom\":[],\"Left\":[{\"id\":\"CS\",\"label\":\"CS\",\"type\":\"input\"},{\"id\":\"A\",\"label\":\"A\",\"type\":\"subsea.ss_hydraulic\"}],\"Right\":[{\"id\":\"B\",\"label\":\"B\",\"type\":\"subsea.ss_hydraulic\"}],\"Top\":[]}"
  Z-011A DN 350 : Lookup_n-D  NumberOfTableDimensions=1  BreakpointsForDimension1=[0 20 30 40 50 60 70 80 90]  BreakpointsForDimension2=[1:3]  Table=[0 399 488 1070 2110 3590 5480 7760 10400]  InternalRulePriority=Speed  RndMeth=Simplest  InputSameDT=on
  Variable kv Hydraulic Flow Element1 : PMIOPort  Side=Left
  Variable kv Hydraulic Flow Element2 : PMIOPort  Port=2  Side=Right
  wires:
  Transfer Fcn2/1 -> Z-011A DN 350/1
  Z-011A DN 350/1 -> Simulink-PS Converter4/1
  Rate Transition1/1 -> ?  "Valve2 opening"
  In1/1 -> Rate Transition1/1, Transfer Fcn2/1
  connections:
  Variable kv Hydraulic Flow Element/LConn2 -- Variable kv Hydraulic Flow Element1/RConn1
  Simulink-PS Converter4/RConn1 -- Variable kv Hydraulic Flow Element/LConn1
  Variable kv Hydraulic Flow Element/RConn1 -- Variable kv Hydraulic Flow Element2/RConn1

== system Pump_system_008/Butterfly valve Z2 ==
  In1 : Inport
  Rate Transition1 : RateTransition  OutPortSampleTime=1
  Simulink-PS Converter4 : nesl_utility/Simulink-PS Converter  PhysicalDomain=network_engine_domain  SubClassName=ps_input  LeftPortType=input  RightPortType=output  PseudoPeriodic=off  Frequencies=[]  NoiseDistribution=none  NoiseParameters=[]  Unit=m^3/s  AffineConversion=off  FilteringAndDerivatives=provide  SimscapeFilterOrder=1  InputFilterTimeConstant=0.001  UdotUserProvided=0
      settings: SourceProductBaseCode=MT,SS
  Transfer Fcn2 : TransferFcn  Denominator=[0.5/5 1]
  Variable kv Hydraulic Flow Element : subsea_lib/Valves/Variable kv Hydraulic Flow Element  ss_location=true  kv=1/3600 m^3/s  kv_min=1.3e-6 m^3/s  q_specify=off  q_priority=None  q=0 m^3/s  q_nominal_specify=off  q_nominal_unit=m^3/s  q_nominal_value=1  p_specify=off  p_priority=None  p=0 Pa  p_nominal_specify=off  p_nominal_unit=Pa  p_nominal_value=1
      settings: SourceProductName=Subsea  InternalSimscapePortConfiguration="{\"Bottom\":[],\"Left\":[{\"id\":\"CS\",\"label\":\"CS\",\"type\":\"input\"},{\"id\":\"A\",\"label\":\"A\",\"type\":\"subsea.ss_hydraulic\"}],\"Right\":[{\"id\":\"B\",\"label\":\"B\",\"type\":\"subsea.ss_hydraulic\"}],\"Top\":[]}"
  Z-011A DN 350 : Lookup_n-D  NumberOfTableDimensions=1  BreakpointsForDimension1=[0 20 30 40 50 60 70 80 90]  BreakpointsForDimension2=[1:3]  Table=[0 399 488 1070 2110 3590 5480 7760 10400]  InternalRulePriority=Speed  RndMeth=Simplest  InputSameDT=on
  Variable kv Hydraulic Flow Element1 : PMIOPort  Side=Left
  Variable kv Hydraulic Flow Element2 : PMIOPort  Port=2  Side=Right
  wires:
  Transfer Fcn2/1 -> Z-011A DN 350/1
  Z-011A DN 350/1 -> Simulink-PS Converter4/1
  Rate Transition1/1 -> ?  "Valve3 opening"
  In1/1 -> Rate Transition1/1, Transfer Fcn2/1
  connections:
  Variable kv Hydraulic Flow Element/LConn2 -- Variable kv Hydraulic Flow Element1/RConn1
  Simulink-PS Converter4/RConn1 -- Variable kv Hydraulic Flow Element/LConn1
  Variable kv Hydraulic Flow Element/RConn1 -- Variable kv Hydraulic Flow Element2/RConn1

== system Pump_system_008/Butterfly valve Z4 ==
  In1 : Inport
  Rate Transition1 : RateTransition  OutPortSampleTime=1
  Simulink-PS Converter4 : nesl_utility/Simulink-PS Converter  PhysicalDomain=network_engine_domain  SubClassName=ps_input  LeftPortType=input  RightPortType=output  PseudoPeriodic=off  Frequencies=[]  NoiseDistribution=none  NoiseParameters=[]  Unit=m^3/s  AffineConversion=off  FilteringAndDerivatives=provide  SimscapeFilterOrder=1  InputFilterTimeConstant=0.001  UdotUserProvided=0
      settings: SourceProductBaseCode=MT,SS
  Transfer Fcn2 : TransferFcn  Denominator=[0.5/5 1]
  Variable kv Hydraulic Flow Element : subsea_lib/Valves/Variable kv Hydraulic Flow Element  ss_location=true  kv=1/3600 m^3/s  kv_min=1.3e-6 m^3/s  q_specify=off  q_priority=None  q=0 m^3/s  q_nominal_specify=off  q_nominal_unit=m^3/s  q_nominal_value=1  p_specify=off  p_priority=None  p=0 Pa  p_nominal_specify=off  p_nominal_unit=Pa  p_nominal_value=1
      settings: SourceProductName=Subsea  InternalSimscapePortConfiguration="{\"Bottom\":[],\"Left\":[{\"id\":\"CS\",\"label\":\"CS\",\"type\":\"input\"},{\"id\":\"A\",\"label\":\"A\",\"type\":\"subsea.ss_hydraulic\"}],\"Right\":[{\"id\":\"B\",\"label\":\"B\",\"type\":\"subsea.ss_hydraulic\"}],\"Top\":[]}"
  Z-011A DN 350 : Lookup_n-D  NumberOfTableDimensions=1  BreakpointsForDimension1=[0 20 30 40 50 60 70 80 90]  BreakpointsForDimension2=[1:3]  Table=[0 399 488 1070 2110 3590 5480 7760 10400]  InternalRulePriority=Speed  RndMeth=Simplest  InputSameDT=on
  Variable kv Hydraulic Flow Element1 : PMIOPort  Side=Left
  Variable kv Hydraulic Flow Element2 : PMIOPort  Port=2  Side=Right
  wires:
  Transfer Fcn2/1 -> Z-011A DN 350/1
  Z-011A DN 350/1 -> Simulink-PS Converter4/1
  Rate Transition1/1 -> ?  "Valve5 opening"
  In1/1 -> Rate Transition1/1, Transfer Fcn2/1
  connections:
  Variable kv Hydraulic Flow Element/LConn2 -- Variable kv Hydraulic Flow Element1/RConn1
  Simulink-PS Converter4/RConn1 -- Variable kv Hydraulic Flow Element/LConn1
  Variable kv Hydraulic Flow Element/RConn1 -- Variable kv Hydraulic Flow Element2/RConn1

== system Pump_system_008/Butterfly valve Z5 ==
  In1 : Inport
  Simulink-PS Converter4 : nesl_utility/Simulink-PS Converter  PhysicalDomain=network_engine_domain  SubClassName=ps_input  LeftPortType=input  RightPortType=output  PseudoPeriodic=off  Frequencies=[]  NoiseDistribution=none  NoiseParameters=[]  Unit=m^3/s  AffineConversion=off  FilteringAndDerivatives=provide  SimscapeFilterOrder=1  InputFilterTimeConstant=0.001  UdotUserProvided=0
      settings: SourceProductBaseCode=MT,SS
  Variable kv Hydraulic Flow Element : subsea_lib/Valves/Variable kv Hydraulic Flow Element  ss_location=true  kv=1/3600 m^3/s  kv_min=1.3e-6 m^3/s  q_specify=off  q_priority=None  q=0 m^3/s  q_nominal_specify=off  q_nominal_unit=m^3/s  q_nominal_value=1  p_specify=off  p_priority=None  p=0 Pa  p_nominal_specify=off  p_nominal_unit=Pa  p_nominal_value=1
      settings: SourceProductName=Subsea  InternalSimscapePortConfiguration="{\"Bottom\":[],\"Left\":[{\"id\":\"CS\",\"label\":\"CS\",\"type\":\"input\"},{\"id\":\"A\",\"label\":\"A\",\"type\":\"subsea.ss_hydraulic\"}],\"Right\":[{\"id\":\"B\",\"label\":\"B\",\"type\":\"subsea.ss_hydraulic\"}],\"Top\":[]}"
  Z-011A DN 350 : Lookup_n-D  NumberOfTableDimensions=1  BreakpointsForDimension1=[0 20 30 40 50 60 70 80 90]  BreakpointsForDimension2=[1:3]  Table=[0 399 488 1070 2110 3590 5480 7760 10400]  InternalRulePriority=Speed  RndMeth=Simplest  InputSameDT=on
  Variable kv Hydraulic Flow Element1 : PMIOPort  Side=Left
  Variable kv Hydraulic Flow Element2 : PMIOPort  Port=2  Side=Right
  wires:
  In1/1 -> Z-011A DN 350/1
  Z-011A DN 350/1 -> Simulink-PS Converter4/1
  connections:
  Variable kv Hydraulic Flow Element/LConn2 -- Variable kv Hydraulic Flow Element1/RConn1
  Simulink-PS Converter4/RConn1 -- Variable kv Hydraulic Flow Element/LConn1
  Variable kv Hydraulic Flow Element/RConn1 -- Variable kv Hydraulic Flow Element2/RConn1

== system Pump_system_008/Subsystem ==
  Gain : Gain  Gain=3600
  PS-Simulink Converter5 : nesl_utility/PS-Simulink Converter  PhysicalDomain=network_engine_domain  SubClassName=ps_output  LeftPortType=input  RightPortType=output  PseudoPeriodic=off  Frequencies=[]  Unit=m^3/s  AffineConversion=off
      settings: SourceProductBaseCode=MT,SS
  in : PMIOPort  Side=Left
  Q m3/h : Outport
  wires:
  PS-Simulink Converter5/1 -> Gain/1
  Gain/1 -> Q m3/h/1
  connections:
  PS-Simulink Converter5/LConn1 -- in/RConn1

== system Pump_system_008/Subsystem1 ==
  Gain : Gain  Gain=3600
  PS-Simulink Converter5 : nesl_utility/PS-Simulink Converter  PhysicalDomain=network_engine_domain  SubClassName=ps_output  LeftPortType=input  RightPortType=output  PseudoPeriodic=off  Frequencies=[]  Unit=m^3/s  AffineConversion=off
      settings: SourceProductBaseCode=MT,SS
  in : PMIOPort  Side=Left
  Q m3/h : Outport
  wires:
  Gain/1 -> Q m3/h/1
  PS-Simulink Converter5/1 -> Gain/1
  connections:
  PS-Simulink Converter5/LConn1 -- in/RConn1

== system Pump_system_008/Subsystem10 ==
  In1 : Inport
  power_pipeline : Inport  Port=2
  Display18 : Display
      settings: Decimation=2
  Gain : Gain  Gain=0.1
  Gain1 : Gain  Gain=1000/3600
  Product : Product
  Rate Transition3 : RateTransition  OutPortSampleTime=1
  power_pipeline1 : Outport
  wires:
  Product/1 -> Display18/1, power_pipeline1/1, Rate Transition3/1  "power_pipeline"
  Gain1/1 -> Product/2
  Gain/1 -> Product/1
  In1/1 -> Gain/1
  Rate Transition3/1 -> ?  "Hydraulic power total"
  power_pipeline/1 -> Gain1/1

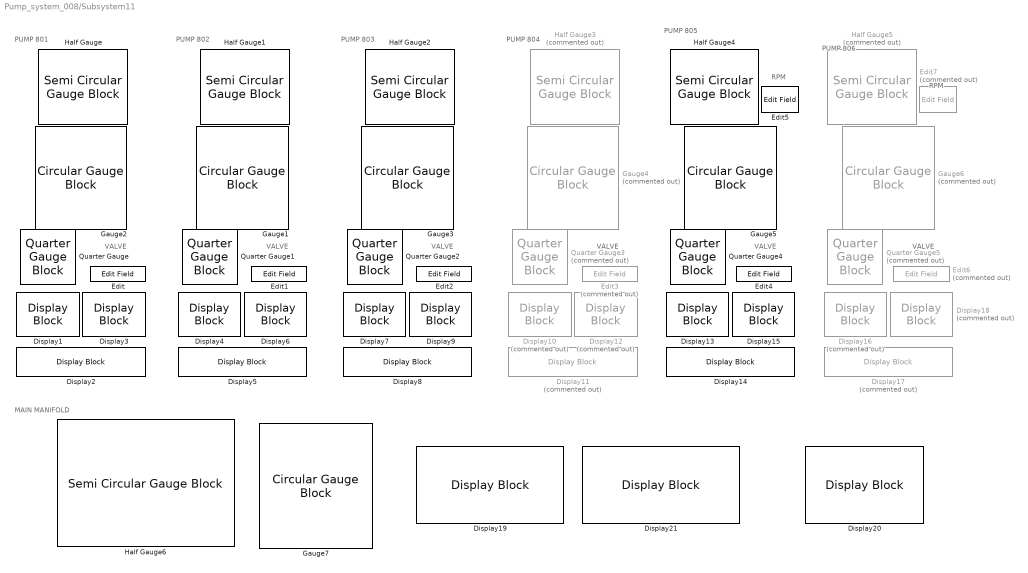
== system Pump_system_008/Subsystem11 ==
  note: PUMP 801
  note: PUMP 802
  note: PUMP 803
  note: PUMP 804
  note: PUMP 805
  note: VALVE
  note: VALVE
  note: VALVE
  note: VALVE
  note: VALVE
  note: RPM
  note: PUMP 806
  note: VALVE
  note: RPM
  note: MAIN MANIFOLD
  Display{1..9,13..15,19..21} (15 alike) : DisplayBlock  Format=Custom  Transparency=1  FormatString=%4.1f
  Display{10..12,16..18} (6 alike) : DisplayBlock  Commented=on  Format=Custom  Transparency=1  FormatString=%4.1f
  Edit{,1..2,4..5} (5 alike) : EditField  LabelPosition=Hide  ShowInitialText=on  Alignment=Center
  Edit3 : EditField  Commented=on  LabelPosition=Hide  ShowInitialText=on  Alignment=Center
  Edit6 : EditField  Commented=on  LabelPosition=Hide  ShowInitialText=on  Alignment=Center
  Edit7 : EditField  Commented=on  LabelPosition=Hide  ShowInitialText=on  Alignment=Center
  Gauge{1..3,5} (4 alike) : CircularGaugeBlock  ScaleMin=4  ScaleMax=10  TickInterval=0.5
  Gauge4 : CircularGaugeBlock  Commented=on  ScaleMin=4  ScaleMax=10  TickInterval=0.5
  Gauge6 : CircularGaugeBlock  Commented=on  ScaleMin=4  ScaleMax=10  TickInterval=0.5
  Gauge7 : CircularGaugeBlock  ScaleMin=5  ScaleMax=6  TickInterval=0.2
  Half Gauge{,1..2,4} (4 alike) : SemiCircularGaugeBlock  ScaleMin=600  ScaleMax=1200
  Half Gauge3 : SemiCircularGaugeBlock  Commented=on  ScaleMin=600  ScaleMax=1200
  Half Gauge5 : SemiCircularGaugeBlock  Commented=on  ScaleMin=600  ScaleMax=1200
  Half Gauge6 : SemiCircularGaugeBlock  ScaleMin=3700  ScaleMax=4500
  Quarter Gauge{,1..2,4} (4 alike) : QuarterGaugeBlock  ScaleMax=90
  Quarter Gauge3 : QuarterGaugeBlock  Commented=on  ScaleMax=90
  Quarter Gauge5 : QuarterGaugeBlock  Commented=on  ScaleMax=90

== system Pump_system_008/Subsystem12 ==
  Pump p : Inport
  RPM : Inport  Port=2
  Pump : Subsystem
  Subsea Hydraulic Flow Source : subsea_lib/Sources/Subsea Hydraulic Flow Source
      settings: SourceProductName=Subsea  InternalSimscapePortConfiguration="{\"Bottom\":[],\"Left\":[{\"id\":\"P\",\"label\":\"P\",\"type\":\"subsea.ss_hydraulic\"}],\"Right\":[{\"id\":\"S\",\"label\":\"S\",\"type\":\"input\"},{\"id\":\"T\",\"label\":\"T\",\"type\":\"subsea.ss_hydraulic\"}],\"Top\":[]}"
  Subsea Hydraulic Flow Source2 : PMIOPort  Side=Left
  Subsea Hydraulic Flow Source1 : PMIOPort  Port=2  Side=Right
  Power : Outport
  wires:
  Pump p/1 -> Pump/2(Pump p)
  RPM/1 -> Pump/1(RPM)
  Pump/1(Power) -> Power/1
  connections:
  Subsea Hydraulic Flow Source/RConn1 -- Pump/RConn1
  Subsea Hydraulic Flow Source/RConn2 -- Subsea Hydraulic Flow Source2/RConn1
  Subsea Hydraulic Flow Source/LConn1 -- Subsea Hydraulic Flow Source1/RConn1

== system Pump_system_008/Subsystem15 ==
  Gain : Gain  Gain=3600
  PS-Simulink Converter5 : nesl_utility/PS-Simulink Converter  PhysicalDomain=network_engine_domain  SubClassName=ps_output  LeftPortType=input  RightPortType=output  PseudoPeriodic=off  Frequencies=[]  Unit=m^3/s  AffineConversion=off
      settings: SourceProductBaseCode=MT,SS
  in : PMIOPort  Side=Left
  Q m3/h : Outport
  wires:
  Gain/1 -> Q m3/h/1
  PS-Simulink Converter5/1 -> Gain/1
  connections:
  PS-Simulink Converter5/LConn1 -- in/RConn1

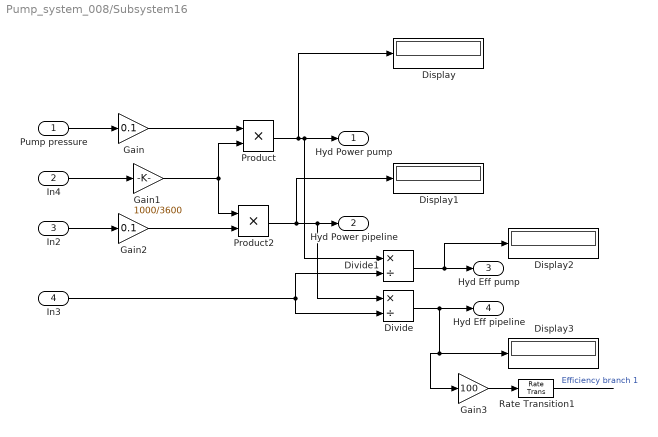
== system Pump_system_008/Subsystem16 ==
  Pump pressure : Inport
  In4 : Inport  Port=2
  In2 : Inport  Port=3
  In3 : Inport  Port=4
  Display{,1..3} (4 alike) : Display
      settings: Decimation=2
  Divide : Product  Inputs=*/
  Divide1 : Product  Inputs=*/
  Gain : Gain  Gain=0.1
  Gain1 : Gain  Gain=1000/3600
  Gain2 : Gain  Gain=0.1
  Gain3 : Gain  Gain=100
  Product : Product
  Product2 : Product
  Rate Transition1 : RateTransition  OutPortSampleTime=1
  Hyd Power pump : Outport
  Hyd Power pipeline : Outport  Port=2
  Hyd Eff pump : Outport  Port=3
  Hyd Eff pipeline : Outport  Port=4
  wires:
  In2/1 -> Gain2/1
  Product/1 -> Display/1, Divide1/1, Hyd Power pump/1
  In4/1 -> Gain1/1
  In3/1 -> Divide1/2, Divide/2
  Pump pressure/1 -> Gain/1
  Gain/1 -> Product/1
  Gain1/1 -> Product/2, Product2/1
  Gain2/1 -> Product2/2
  Product2/1 -> Divide/1, Hyd Power pipeline/1, Display1/1
  Divide1/1 -> Display2/1, Hyd Eff pump/1
  Divide/1 -> Hyd Eff pipeline/1, Display3/1, Gain3/1
  Rate Transition1/1 -> ?  "Efficiency branch 1"
  Gain3/1 -> Rate Transition1/1
